simulink model "spr_sim"  (R2023b)
settings: Solver=ode23tb  StartTime=0.0  StopTime=inf  MaxStep=100e-6  RelTol=1e-3
values from neighbouring files (symbols this model uses):
  alfa = 0    [spr.m]
  f = 50    [spr.m]
  L_obc = 100e-6    (= 0.0001)    [spr.m]
  Lin = 100e-6    (= 0.0001)    [spr.m]
  Ls = 50e-6    (= 5e-05)    [spr.m]
  R_obc = 6    [spr.m]
  Rin = 1/30*w*Lin    (= 0.0010471975512)    [spr.m]
  Us_ab = 400    [spr.m]
undefined symbols (not defined in the file or in its folder): D1, lagging, pulse
libraries: spsSeriesRLCBranchLib x7, spsThyristorLib x6, spsThreePhaseVIMeasurementLib x2, spsCurrentMeasurementLib x1, spsGroundLib x1, spsPLL3phLib x1, spsPulseGeneratorThyristor6PulseLib x1, spsThreePhaseProgrammableVoltageSourceLib x1, spsVoltageMeasurementLib x1, spspowerguiLib x1
settings Model: SimulationMode=accelerator  Creator=Fortis  LastModifiedBy=rolni
settings DataIOCC: ReturnWorkspaceOutputs=off

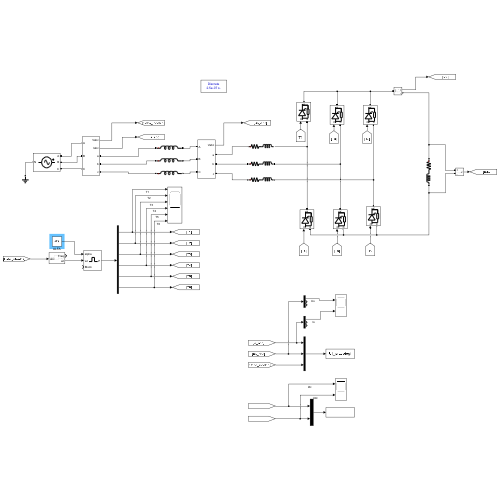
[thumbnail: Simulink's stored preview of the top-level diagram]
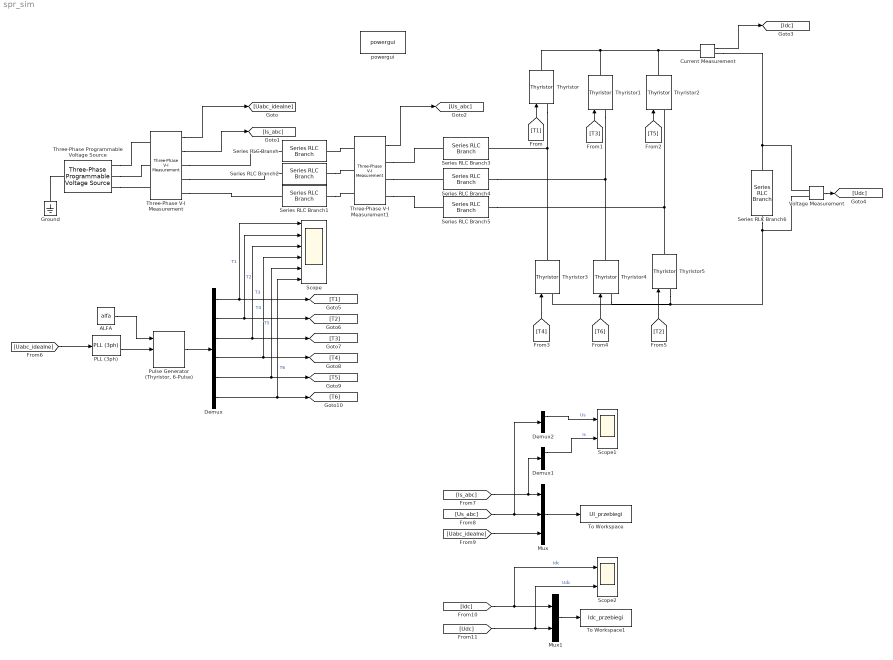
== system spr_sim ==
  ALFA : Constant  Value=alfa
  Current Measurement : spsCurrentMeasurementLib/Current Measurement  PhasorSimulation=off  OutputType=Complex  PSBequivalent=0
  Demux : Demux  Outputs=6
  Demux1 : Demux  Outputs=3
  Demux2 : Demux  Outputs=3
  Ground : spsGroundLib/Ground  LConnTagsString=a
  Mux : Mux  Inputs=3
  Mux1 : Mux  Inputs=2
  PLL (3ph) : spsPLL3phLib/PLL (3ph)  Fmin=45  Par_Init=[0, f]  ParK=[180, 3200, 1]  TcD=1e-4  MaxRateChangeFreq=12  FilterCutOffFreq=25  Ts=0  AGC=on
  "Pulse Generator (Thyristor, 6-Pulse)" : spsPulseGeneratorThyristor6PulseLib/Pulse Generator (Thyristor, 6-Pulse)  GenType=6-pulse  Delta=D1 (lagging)  pwidth=5  Double_Pulse=on  Ts=0
      settings: LibrarySourceBlock=|
      | sps_lib/Power Electronics/Power Electronics Control/Pulse Generator
      | (Thyristor, 6-Pulse)
  Scope : Scope  NumInputPorts=6
  Scope1 : Scope  NumInputPorts=2
  Scope2 : Scope  NumInputPorts=2
  Series RLC Branch : spsSeriesRLCBranchLib/Series RLC Branch  LConnTagsString=__new0  RConnTagsString=__new0  BranchType=L  Resistance=1  Inductance=Ls  SetiL0=off  InitialCurrent=0  Capacitance=1e-6  Setx0=off  InitialVoltage=0  Measurements=None
  Series RLC Branch1 : spsSeriesRLCBranchLib/Series RLC Branch  LConnTagsString=__new0  RConnTagsString=__new0  BranchType=L  Resistance=1  Inductance=Ls  SetiL0=off  InitialCurrent=0  Capacitance=1e-6  Setx0=off  InitialVoltage=0  Measurements=None
  Series RLC Branch2 : spsSeriesRLCBranchLib/Series RLC Branch  LConnTagsString=__new0  RConnTagsString=__new0  BranchType=L  Resistance=1  Inductance=Ls  SetiL0=off  InitialCurrent=0  Capacitance=1e-6  Setx0=off  InitialVoltage=0  Measurements=None
  Series RLC Branch3 : spsSeriesRLCBranchLib/Series RLC Branch  LConnTagsString=__new0  RConnTagsString=__new0  BranchType=RL  Resistance=Rin  Inductance=Lin  SetiL0=off  InitialCurrent=0  Capacitance=1e-6  Setx0=off  InitialVoltage=0  Measurements=None
  Series RLC Branch4 : spsSeriesRLCBranchLib/Series RLC Branch  LConnTagsString=__new0  RConnTagsString=__new0  BranchType=RL  Resistance=Rin  Inductance=Lin  SetiL0=off  InitialCurrent=0  Capacitance=1e-6  Setx0=off  InitialVoltage=0  Measurements=None
  Series RLC Branch5 : spsSeriesRLCBranchLib/Series RLC Branch  LConnTagsString=__new0  RConnTagsString=__new0  BranchType=RL  Resistance=Rin  Inductance=Lin  SetiL0=off  InitialCurrent=0  Capacitance=1e-6  Setx0=off  InitialVoltage=0  Measurements=None
  Series RLC Branch6 : spsSeriesRLCBranchLib/Series RLC Branch  LConnTagsString=__new0  RConnTagsString=__new0  BranchType=RL  Resistance=R_obc  Inductance=L_obc  SetiL0=off  InitialCurrent=0  Capacitance=1e-6  Setx0=off  InitialVoltage=0  Measurements=None
  Three-Phase Programmable Voltage Source : spsThreePhaseProgrammableVoltageSourceLib/Three-Phase Programmable Voltage Source  PositiveSequence="[Us_ab  fi f]"  VariationEntity=None  VariationType=Table of time-amplitude pairs  VariationTypeAlt=Step  VariationStep=0.5  VariationRate=10  VariationMagnitude=0.3  VariationFrequency=2  VariationTiming=[1 2]  VariationPhaseA=off  Amplitudes=[1 0.8 1.2 1.0]  TimeValues=[0 0.1 0.15 0.2]  HarmonicGeneration=off  HarmonicA=[3 0.2 -25 0]  HarmonicB=[2 0.15 35 2]  Timing="[0.05  3]"  BusType=swing  Pref=0  Qref=0  Qmin=-inf  Qmax=inf
  Three-Phase V-I Measurement : spsThreePhaseVIMeasurementLib/Three-Phase V-I Measurement  VoltageMeasurement=phase-to-ground  SetLabelV=off  LabelV=Vabc  Vpu=off  VpuLL=off  CurrentMeasurement=yes  SetLabelI=off  LabelI=Iabc  Ipu=off  Pbase=100e6  Vbase=500e3  OutputType=Complex  PhasorSimulation=off  PSBequivalent=0
  Three-Phase V-I Measurement1 : spsThreePhaseVIMeasurementLib/Three-Phase V-I Measurement  VoltageMeasurement=phase-to-ground  SetLabelV=off  LabelV=Vabc  Vpu=off  VpuLL=off  CurrentMeasurement=no  SetLabelI=off  LabelI=Iabc  Ipu=off  Pbase=100e6  Vbase=500e3  OutputType=Complex  PhasorSimulation=off  PSBequivalent=0
  Thyristor{,1..5} (6 alike) : spsThyristorLib/Thyristor  Ron=Rdiode  Lon=0  Vf=Vdiode  IC=0  Rs=500  Cs=250e-9  Measurements=off
  To Workspace : ToWorkspace  VariableName=UI_przebiegi  SaveFormat=Structure With Time  SampleTime=-1
  To Workspace1 : ToWorkspace  VariableName=Idc_przebiegi  SaveFormat=Structure With Time  SampleTime=-1
  Voltage Measurement : spsVoltageMeasurementLib/Voltage Measurement  PhasorSimulation=off  OutputType=Complex  PSBequivalent=0
  powergui : spspowerguiLib/powergui  Priority=1  SimulationMode=Discrete  SampleTime=2.5e-07  frequency=60  Iterations=50  frequencyindice=50  Pbase=100e6  ErrMax=1e-4  UnitsV=kV  UnitsW=MW  buscounter=0  FunctionMessages=off  echomessages=off  EnableUseOfTLC=off  CurrentSourceSwitches=off  DisableSnubberDevices=off  DisableRonSwitches=off  DisableVfSwitches=off  DisplayEquations=off  AutomaticDiscreteSolvers=off  SolverType=Tustin/Backward Euler (TBE)  Interpol=off  ExternalGateDelay=off  methode=off  Ts=100  x0status=blocks  SPID=on  SwTol=0  HookPort=off  NonlinearTolerance=1e-4  nMaxIteration=100  ContinueOnMaxIteration=off  RestoreLinks=warning  ResistiveCurrentMeasurement=off  Frange=[0:2:500]  Ylog=off  Xlog=on  ShowGrid=off  save=off  variable=ZData  structure=0  ZoomFFT=off  StartTime=0.0  cycles=1  DisplayStyle=1  fundamental=60  FreqAxis=off  MaxFrequency=1000  frequencyindicesteady=1  RmsSteady=1  display=off
  wires:
  Three-Phase V-I Measurement/1 -> [Uabc_idealne]
  Three-Phase V-I Measurement/2 -> [Is_abc]
  Three-Phase V-I Measurement1/1 -> [Us_abc]
  [T1] -> Thyristor/1
  [T4] -> Thyristor3/1
  [T6] -> Thyristor4/1
  [T2] -> Thyristor5/1
  Current Measurement/1 -> [Idc]
  Voltage Measurement/1 -> [Udc]
  [Uabc_idealne] -> PLL (3ph)/1
  PLL (3ph)/2 -> "Pulse Generator (Thyristor, 6-Pulse)"/2
  ALFA/1 -> "Pulse Generator (Thyristor, 6-Pulse)"/1
  "Pulse Generator (Thyristor, 6-Pulse)"/1 -> Demux/1
  Demux/1 -> Scope/1, [T1]  "T1"
  Demux/2 -> Scope/2, [T2]  "T2"
  Demux/3 -> Scope/3, [T3]  "T3"
  Demux/4 -> Scope/4, [T4]  "T4"
  Demux/5 -> Scope/5, [T5]  "T5"
  Demux/6 -> Scope/6, [T6]  "T6"
  [Is_abc] -> Demux1/1, Mux/1
  [Us_abc] -> Demux2/1, Mux/2
  [Uabc_idealne] -> Mux/3
  Mux/1 -> To Workspace/1
  Demux2/1 -> Scope1/1  "Us"
  Demux1/1 -> Scope1/2  "Is"
  [Idc] -> Scope2/1, Mux1/1  "Idc"
  [Udc] -> Scope2/2, Mux1/2  "Udc"
  Mux1/1 -> To Workspace1/1
  [T3] -> Thyristor1/1
  [T5] -> Thyristor2/1
  connections:
  Three-Phase V-I Measurement/RConn1 -- Series RLC Branch/LConn1
  Three-Phase V-I Measurement/RConn2 -- Series RLC Branch2/LConn1
  Three-Phase V-I Measurement/RConn3 -- Series RLC Branch1/LConn1
  Three-Phase V-I Measurement1/LConn1 -- Series RLC Branch/RConn1
  Series RLC Branch2/RConn1 -- Three-Phase V-I Measurement1/LConn2
  Series RLC Branch1/RConn1 -- Three-Phase V-I Measurement1/LConn3
  Three-Phase Programmable Voltage Source/RConn1 -- Three-Phase V-I Measurement/LConn1
  Three-Phase Programmable Voltage Source/RConn2 -- Three-Phase V-I Measurement/LConn2
  Three-Phase Programmable Voltage Source/RConn3 -- Three-Phase V-I Measurement/LConn3
  Three-Phase Programmable Voltage Source/LConn1 -- Ground/LConn1
  Three-Phase V-I Measurement1/RConn1 -- Series RLC Branch3/LConn1
  Three-Phase V-I Measurement1/RConn2 -- Series RLC Branch4/LConn1
  Three-Phase V-I Measurement1/RConn3 -- Series RLC Branch5/LConn1
  Thyristor/LConn1 -- Thyristor3/RConn1 -- Series RLC Branch3/RConn1
  Series RLC Branch4/RConn1 -- Thyristor4/RConn1 -- Thyristor1/LConn1
  Series RLC Branch5/RConn1 -- Thyristor2/LConn1 -- Thyristor5/RConn1
  Thyristor/RConn1 -- Thyristor1/RConn1 -- Thyristor2/RConn1 -- Current Measurement/LConn1
  Current Measurement/RConn1 -- Voltage Measurement/LConn1 -- Series RLC Branch6/LConn1
  Series RLC Branch6/RConn1 -- Voltage Measurement/LConn2 -- Thyristor5/LConn1 -- Thyristor4/LConn1 -- Thyristor3/LConn1
